simulink model "tp2_2"  (R2023b)
settings: Solver=VariableStepAuto  StartTime=0.0  StopTime=50.0  RelTol=1e-3
settings Model: Creator=rusha  LastModifiedBy=rusha

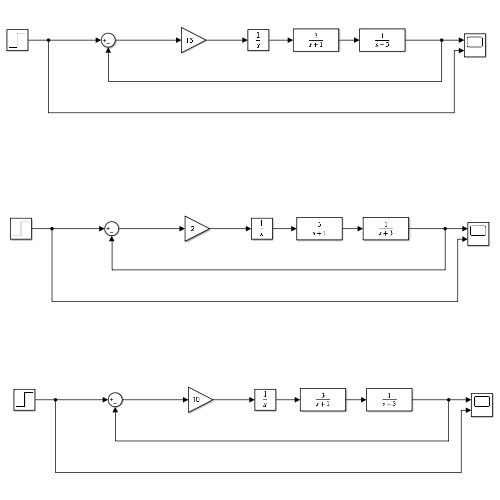
[thumbnail: Simulink's stored preview of the top-level diagram]
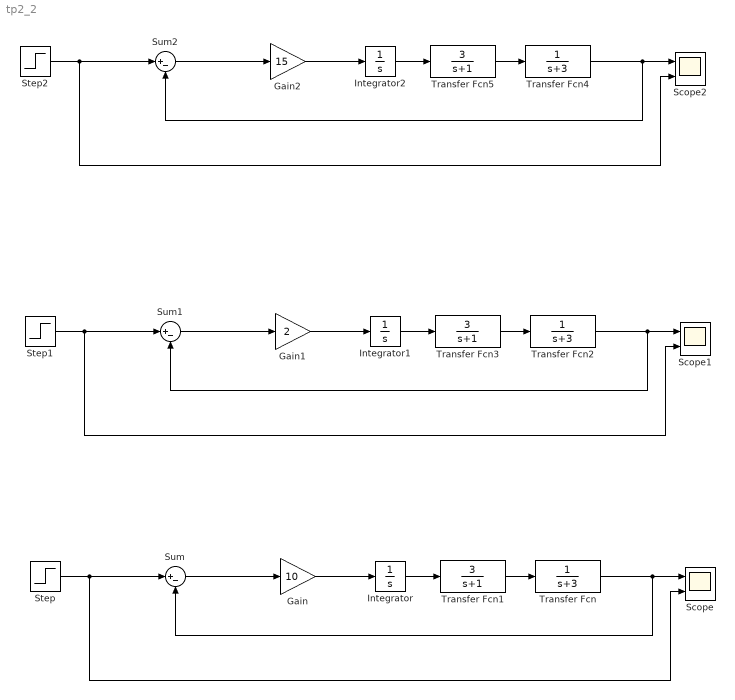
== system tp2_2 ==
  Gain : Gain  Gain=10
  Gain1 : Gain  Gain=2
  Gain2 : Gain  Gain=15
  Integrator : Integrator
  Integrator1 : Integrator
  Integrator2 : Integrator
  Scope : Scope  NumInputPorts=2
  Scope1 : Scope  NumInputPorts=2
  Scope2 : Scope  NumInputPorts=2
  Step : Step  SampleTime=0
  Step1 : Step  SampleTime=0
  Step2 : Step  SampleTime=0
  Sum : Sum  Inputs=|+-
  Sum1 : Sum  Inputs=|+-
  Sum2 : Sum  Inputs=|+-
  Transfer Fcn : TransferFcn  Denominator=[1 3]
  Transfer Fcn1 : TransferFcn  Numerator=[3]  Denominator=[1 1]
  Transfer Fcn2 : TransferFcn  Denominator=[1 3]
  Transfer Fcn3 : TransferFcn  Numerator=[3]  Denominator=[1 1]
  Transfer Fcn4 : TransferFcn  Denominator=[1 3]
  Transfer Fcn5 : TransferFcn  Numerator=[3]  Denominator=[1 1]
  wires:
  Transfer Fcn1/1 -> Transfer Fcn/1
  Transfer Fcn/1 -> Sum/2, Scope/1
  Step/1 -> Scope/2, Sum/1
  Sum/1 -> Gain/1
  Integrator/1 -> Transfer Fcn1/1
  Gain/1 -> Integrator/1
  Transfer Fcn3/1 -> Transfer Fcn2/1
  Sum1/1 -> Gain1/1
  Gain1/1 -> Integrator1/1
  Step1/1 -> Scope1/2, Sum1/1
  Integrator1/1 -> Transfer Fcn3/1
  Transfer Fcn2/1 -> Sum1/2, Scope1/1
  Transfer Fcn5/1 -> Transfer Fcn4/1
  Sum2/1 -> Gain2/1
  Gain2/1 -> Integrator2/1
  Step2/1 -> Scope2/2, Sum2/1
  Integrator2/1 -> Transfer Fcn5/1
  Transfer Fcn4/1 -> Sum2/2, Scope2/1
